simulink model "IFM_ModelComposer"  (R2024b)
settings: Solver=VariableStepAuto  StartTime=0.0  StopTime=2e-4  RelTol=1e-3
PreLoadFcn:
  | System
values from neighbouring files (symbols this model uses):
  Fs = 300e6    (= 300000000)    [IFM.m]    (also in System.m; SystemInput.m = p.Results.Fs)
  JustNoiseSamples = Fs*JustNoiseTime    (= 30000)    [IFM.m]    (also in System.m; SystemInput.m = Fs * 100e-6)
undefined symbols (not defined in the file or in its folder): IFM, Trial
libraries: hdlBasic x91, hdlDSPIP x2, vmcUtilities x1
settings Model: Creator=fsy  LastModifiedBy=fsy

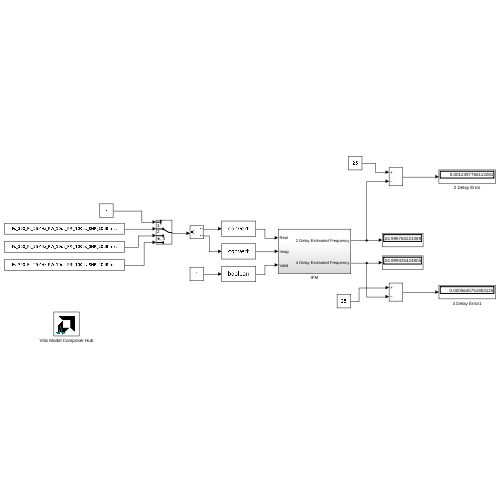
[thumbnail: Simulink's stored preview of the top-level diagram]
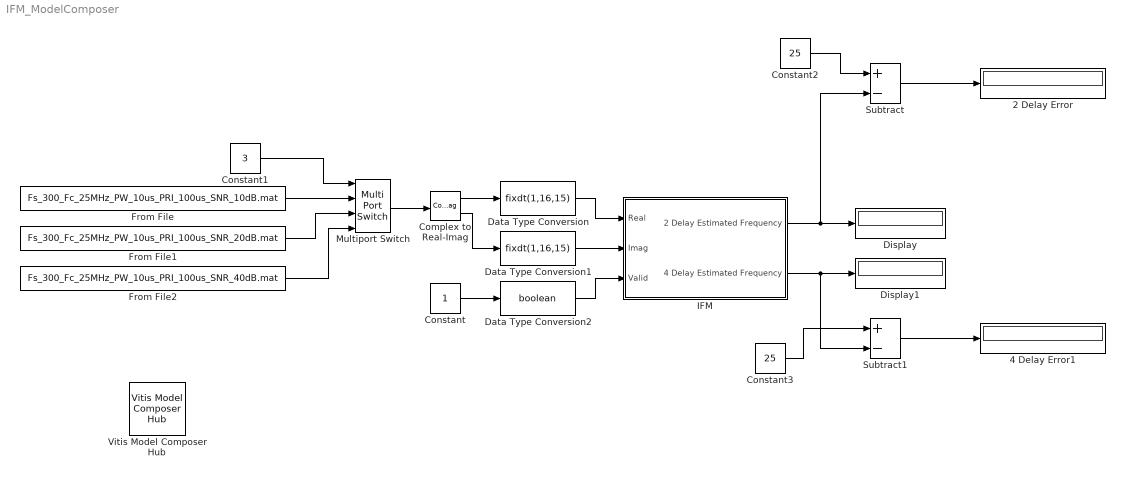
== system IFM_ModelComposer ==
  2 Delay Error : Display
  4 Delay Error1 : Display
  Complex to Real-Imag : ComplexToRealImag
  Constant : Constant  SampleTime=1/Fs
  Constant1 : Constant  Value=3  SampleTime=1/Fs
  Constant2 : Constant  Value=25  SampleTime=1/Fs
  Constant3 : Constant  Value=25  SampleTime=1/Fs
  Data Type Conversion : DataTypeConversion  OutDataTypeStr=fixdt(1,16,15)  RndMeth=Round
  Data Type Conversion1 : DataTypeConversion  OutDataTypeStr=fixdt(1,16,15)  RndMeth=Round
  Data Type Conversion2 : DataTypeConversion  OutDataTypeStr=boolean  RndMeth=Round
  Display : Display
  Display1 : Display
  From File : FromFile  FileName=Fs_300_Fc_25MHz_PW_10us_PRI_100us_SNR_10dB.mat  SampleTime=1/Fs
  From File1 : FromFile  FileName=Fs_300_Fc_25MHz_PW_10us_PRI_100us_SNR_20dB.mat  SampleTime=1/Fs
  From File2 : FromFile  FileName=Fs_300_Fc_25MHz_PW_10us_PRI_100us_SNR_40dB.mat  SampleTime=1/Fs
  IFM : Subsystem
  Multiport Switch : MultiPortSwitch  OutDataTypeStr=double  SaturateOnIntegerOverflow=off  InputSameDT=off
  Subtract : Sum  Inputs=+-
  Subtract1 : Sum  Inputs=+-
  Vitis Model Composer Hub : vmcUtilities/Vitis Model Composer Hub  Tag=genX  CodeGeneration=off  SubsystemName=IFM  BlockHierPath=Trial/IFM  CompilationType=HDLCompilation  SubsystemType=HDLNode  ExportTypeV2=IP Catalog  StartColumn=1  NumberOfColumns=1  TargetDirectory=./netlist\ip\IFM\src  exportDesign=off  analyzeDesign=on  validateDesignOnHw=off  ExportType=AI Engines  IpVendor=xilinx.com  IpLibrary=hls  IpVersion=1.0  IpHWLanguage=Verilog  AieCompilerOptions={}  AieSimulatorOptions={}  CreateTestbench=on  TestbenchStackSize=10  RunRtlSim=off  RunCSim=off  RunAieSim=off  AieSimTimeout=50000  RunAieSimProfiling=off  LaunchVitisAnalyzer=off  PlotOutput=off  RunX86Sim=off  X86SimTimeout=10  GenHwImage=off  GenLibadfXo=on  GenHwValidationCode=off  PlatformType=Not Specified  HwSystemType=Baremetal  HwValidationTarget=hw  ProjDevice=Zynq UltraScale+ ZCU102 Evaluation Board (xczu9eg-ffvb1156-2-e)  ProjDevicePart=xczu9eg-ffvb1156-2-e  AIEType=None  SamplePeriod=-1  ClockFrequency=200  DataPathParallelism=1  xilinxfamily=zynquplus  part=xczu9eg  speed=-2-e  package=ffvb1156  directory=./netlist\ip\IFM\src  testbench=off  incr_netlist=off  synthesis_tool=Vivado  clock_wrapper=Clock Enables  dbl_ovrd=According to Block Masks  dcm_input_clock_period=10  sysclk_period=1e9/Fs  simulink_period=1/Fs  eval_field=0  IPInfoJsonString="{\"DUTSubsystemName\":\"IFM\",\"HDLSubsystem\":{\"SubsystemName\":\"IFM\",\"IPName\":\"Subsystem\",\"IPLibrary\":\"VMC\",\"IPVendor\":\"User Company\",\"IPVersion\":\"1.0\",\"TargetDirectory\":\"./netlist\",\"SubsystemDir\":\"./netlist\\\\ip\\\\IFM\",\"FreqHz\":\"300000000\"},\"SubsystemTag\":\"HDLNode\"}"  LogFileName=C:\Users\fsydere\Workspace\IFM\Model Composer\netlist\model_composer.log  NThreads=4  IPConfigFile=C:\Users\fsydere\AppData\Local\Temp\vmctmp-13469454594715593076\Trial_ipconfig.json
  wires:
  Subtract/1 -> 2 Delay Error/1
  IFM/2(4 Delay Estimated Frequency) -> Subtract1/2, Display1/1
  IFM/1(2 Delay Estimated Frequency) -> Subtract/2, Display/1
  Data Type Conversion1/1 -> IFM/2(Imag)
  Data Type Conversion2/1 -> IFM/3(Valid)
  Data Type Conversion/1 -> IFM/1(Real)
  Complex to Real-Imag/2 -> Data Type Conversion1/1
  Constant/1 -> Data Type Conversion2/1
  Constant1/1 -> Multiport Switch/1
  Subtract1/1 -> 4 Delay Error1/1
  From File/1 -> Multiport Switch/2
  Multiport Switch/1 -> Complex to Real-Imag/1
  From File1/1 -> Multiport Switch/3
  Complex to Real-Imag/1 -> Data Type Conversion/1
  From File2/1 -> Multiport Switch/4
  Constant3/1 -> Subtract1/1
  Constant2/1 -> Subtract/1

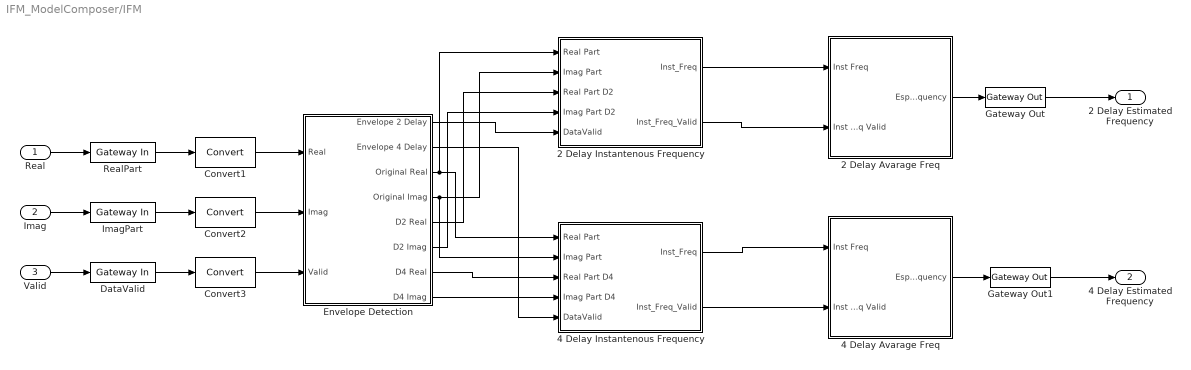
== system IFM_ModelComposer/IFM ==
  Real : Inport
  Imag : Inport  Port=2
  Valid : Inport  Port=3
  2 Delay Avarage Freq : Subsystem
  2 Delay Instantenous Frequency : Subsystem
  4 Delay Avarage Freq : Subsystem
  4 Delay Instantenous Frequency : Subsystem
  Convert1 : hdlBasic/Convert  gui_display_data_type=Fixed-point  arith_type="Signed  (2's comp)"  n_bits=16  bin_pt=15  float_type=Single  exp_bits=8  fraction_bits=24  quantization=Truncate  overflow=Wrap  en=off  latency=0  pipeline=off  XmcBlockStatus=1  maskContainerNames=group2  block_type=convert  block_config=sysgen:Convert_config  block_width=595  block_height=885
  Convert2 : hdlBasic/Convert  gui_display_data_type=Fixed-point  arith_type="Signed  (2's comp)"  n_bits=16  bin_pt=15  float_type=Single  exp_bits=8  fraction_bits=24  quantization=Truncate  overflow=Wrap  en=off  latency=0  pipeline=off  XmcBlockStatus=1  maskContainerNames=group2  block_type=convert  block_config=sysgen:Convert_config  block_width=595  block_height=885
  Convert3 : hdlBasic/Convert  gui_display_data_type=Boolean  arith_type=Boolean  n_bits=16  bin_pt=15  float_type=Single  exp_bits=8  fraction_bits=24  quantization=Truncate  overflow=Wrap  en=off  latency=0  pipeline=off  XmcBlockStatus=1  maskContainerNames=group2  block_type=convert  block_config=sysgen:Convert_config  block_width=595  block_height=885
  DataValid : hdlBasic/Gateway In  gui_display_data_type=Boolean  arith_type=Boolean  n_bits=16  bin_pt=15  preci_type=Single  exp_width=8  frac_width=24  rows=1  columns=1  quantization="Round  (unbiased: +/- Inf)"  overflow=Saturate  period=1/Fs  UseAsADC=off  ADCChannel='1'  interface=None  automatic_assignment=on  address_offset=hex2dec('00')  intf_name=''  intf_description=''  default_value=0  timing_constraint=None  locs_specified=off  LOCs={}  io_standard={}  inherit_from_input=off  hdl_port=on  XmcBlockStatus=1  maskContainerNames=group4  block_type=gatewayin  block_config=sysgen:gateway_in_config  block_width_w=590  block_height_w=620  block_width=640  block_height=850
  Envelope Detection : Subsystem
  Gateway Out : hdlBasic/Gateway Out  inherit_from_input=on  bool_to_boolean=off  hdl_port=off  rows=1  columns=1  UseAsDAC=off  DACChannel='1'  interface=None  automatic_assignment=on  address_offset=hex2dec('00')  intf_name=''  intf_description=''  timing_constraint=None  locs_specified=off  LOCs={}  io_standard={}  XmcBlockStatus=1  maskContainerNames=group4  block_type=gatewayout  block_config=sysgen:gateway_out_config  block_width_w=590  block_height_w=620  block_width=620  block_height=750
  Gateway Out1 : hdlBasic/Gateway Out  inherit_from_input=on  bool_to_boolean=off  hdl_port=off  rows=1  columns=1  UseAsDAC=off  DACChannel='1'  interface=None  automatic_assignment=on  address_offset=hex2dec('00')  intf_name=''  intf_description=''  timing_constraint=None  locs_specified=off  LOCs={}  io_standard={}  XmcBlockStatus=1  maskContainerNames=group4  block_type=gatewayout  block_config=sysgen:gateway_out_config  block_width_w=590  block_height_w=620  block_width=620  block_height=750
  ImagPart : hdlBasic/Gateway In  gui_display_data_type=Fixed-point  arith_type=Signed (2's comp)  n_bits=16  bin_pt=15  preci_type=Single  exp_width=8  frac_width=24  rows=1  columns=1  quantization=Truncate  overflow=Wrap  period=1/Fs  UseAsADC=off  ADCChannel='1'  interface=None  automatic_assignment=on  address_offset=hex2dec('00')  intf_name=''  intf_description=''  default_value=0  timing_constraint=None  locs_specified=off  LOCs={}  io_standard={}  inherit_from_input=off  hdl_port=on  XmcBlockStatus=1  maskContainerNames=group4  block_type=gatewayin  block_config=sysgen:gateway_in_config  block_width_w=590  block_height_w=620  block_width=640  block_height=850
  RealPart : hdlBasic/Gateway In  gui_display_data_type=Fixed-point  arith_type=Signed (2's comp)  n_bits=16  bin_pt=15  preci_type=Single  exp_width=8  frac_width=24  rows=1  columns=1  quantization=Truncate  overflow=Wrap  period=1/Fs  UseAsADC=off  ADCChannel='1'  interface=None  automatic_assignment=on  address_offset=hex2dec('00')  intf_name=''  intf_description=''  default_value=0  timing_constraint=None  locs_specified=off  LOCs={}  io_standard={}  inherit_from_input=off  hdl_port=on  XmcBlockStatus=1  maskContainerNames=group4  block_type=gatewayin  block_config=sysgen:gateway_in_config  block_width_w=590  block_height_w=620  block_width=640  block_height=850
  2 Delay Estimated Frequency : Outport
  4 Delay Estimated Frequency : Outport  Port=2
  wires:
  Real/1 -> RealPart/1
  Valid/1 -> DataValid/1
  Imag/1 -> ImagPart/1
  RealPart/1 -> Convert1/1
  ImagPart/1 -> Convert2/1
  Convert2/1 -> Envelope Detection/2(Imag)
  Convert1/1 -> Envelope Detection/1(Real)
  Envelope Detection/6(D2 Imag) -> 2 Delay Instantenous Frequency/4(Imag Part D2)
  DataValid/1 -> Convert3/1
  Convert3/1 -> Envelope Detection/3(Valid)
  Envelope Detection/1(Envelope 2 Delay) -> 2 Delay Instantenous Frequency/5(DataValid)
  Envelope Detection/5(D2 Real) -> 2 Delay Instantenous Frequency/3(Real Part D2)
  Envelope Detection/2(Envelope 4 Delay) -> 4 Delay Instantenous Frequency/5(DataValid)
  Envelope Detection/3(Original Real) -> 2 Delay Instantenous Frequency/1(Real Part), 4 Delay Instantenous Frequency/1(Real Part)
  Envelope Detection/4(Original Imag) -> 2 Delay Instantenous Frequency/2(Imag Part), 4 Delay Instantenous Frequency/2(Imag Part)
  Envelope Detection/7(D4 Real) -> 4 Delay Instantenous Frequency/3(Real Part D4)
  Envelope Detection/8(D4 Imag) -> 4 Delay Instantenous Frequency/4(Imag Part D4)
  2 Delay Instantenous Frequency/1(Inst_Freq) -> 2 Delay Avarage Freq/1(Inst Freq)
  2 Delay Instantenous Frequency/2(Inst_Freq_Valid) -> 2 Delay Avarage Freq/2(Inst Freq Valid)
  4 Delay Instantenous Frequency/1(Inst_Freq) -> 4 Delay Avarage Freq/1(Inst Freq)
  4 Delay Instantenous Frequency/2(Inst_Freq_Valid) -> 4 Delay Avarage Freq/2(Inst Freq Valid)
  4 Delay Avarage Freq/1(Espected Frequency) -> Gateway Out1/1
  2 Delay Avarage Freq/1(Espected Frequency) -> Gateway Out/1
  Gateway Out/1 -> 2 Delay Estimated Frequency/1
  Gateway Out1/1 -> 4 Delay Estimated Frequency/1

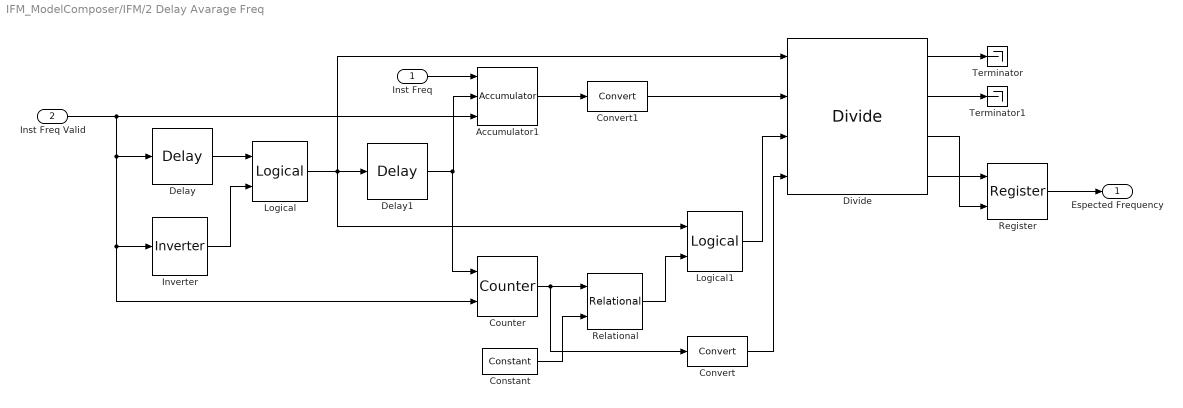
== system IFM_ModelComposer/IFM/2 Delay Avarage Freq ==
  Inst Freq : Inport
  Inst Freq Valid : Inport  Port=2
  Accumulator1 : hdlBasic/Accumulator  operation=Add  n_bits=64  overflow=Wrap  scale=1  rst=on  hasbypass=off  en=on  latency=1  msb_inp=100  msb=100  lsb=-100  use_behavioral_HDL=on  implementation=Fabric  XmcBlockStatus=1  maskContainerNames=group3  block_type=accum  block_config=sysgen:Accum_config  block_width=566  block_height=845
  Constant : hdlBasic/Constant  const=2  gui_display_data_type=Fixed-point  arith_type=Unsigned  n_bits=16  bin_pt=0  preci_type=Single  exp_width=8  frac_width=24  explicit_period=off  period=1  XmcBlockStatus=1  maskContainerNames=tabcontainer1  block_type=constant  block_config=sysgen:Constant_config
  Convert : hdlBasic/Convert  gui_display_data_type=Fixed-point  arith_type="Signed  (2's comp)"  n_bits=64  bin_pt=26  float_type=Single  exp_bits=8  fraction_bits=24  quantization=Truncate  overflow=Wrap  en=off  latency=0  pipeline=off  XmcBlockStatus=1  maskContainerNames=group2  block_type=convert  block_config=sysgen:Convert_config  block_width=595  block_height=885
  Convert1 : hdlBasic/Convert  gui_display_data_type=Fixed-point  arith_type="Signed  (2's comp)"  n_bits=64  bin_pt=26  float_type=Single  exp_bits=8  fraction_bits=24  quantization=Truncate  overflow=Wrap  en=off  latency=0  pipeline=off  XmcBlockStatus=1  maskContainerNames=group2  block_type=convert  block_config=sysgen:Convert_config  block_width=595  block_height=885
  Counter : hdlBasic/Counter  cnt_type=Free running  cnt_to=Inf  operation=Up  start_count=0  cnt_by_val=1  arith_type=Unsigned  n_bits=16  bin_pt=0  load_pin=off  rst=on  en=on  explicit_period=Explicit  period=1/Fs  use_behavioral_HDL=off  implementation=Fabric  XmcBlockStatus=1  maskContainerNames=group1  block_type=counter  block_config=sysgen:Counter_config  block_width=531  block_height=1023
  Delay : hdlBasic/Delay  rst=off  en=off  latency=1  reg_retiming=off  XmcBlockStatus=1  maskContainerNames=group1  block_type=delay  block_config=sysgen:Delay_config
  Delay1 : hdlBasic/Delay  rst=off  en=off  latency=1  reg_retiming=off  XmcBlockStatus=1  maskContainerNames=group1  block_type=delay  block_config=sysgen:Delay_config
  Divide : hdlBasic/Divide  flow_control=Blocking  axi_optimize_goal=Resources  algorithm_type=High_Radix  fractional_width=26  latency=1  rate=1  has_a_tlast=off  has_a_tuser=off  has_b_tlast=off  has_b_tuser=off  en=off  has_result_tready=off  result_tlast_behv=Pass_A_TLAST  has_underflow=off  has_overflow=off  has_invalid_op=off  has_divide_by_zero=off  fpo_op_type=mergeddivide  XmcBlockStatus=1  maskContainerNames=tabcontainer1  block_type=divide  block_config=sysgen:FPOBlockDescriptor_config
  Inverter : hdlBasic/Inverter  en=off  latency=0  XmcBlockStatus=1  maskContainerNames=group2  block_type=inv  block_config=sysgen:Inverter_config
  Logical : hdlBasic/Logical  logical_function=AND  inputs=2  en=off  latency=0  precision=Full  arith_type=Unsigned  n_bits=16  bin_pt=0  align_bp=on  overflow=[]  quantization=[]  XmcBlockStatus=1  maskContainerNames=tabcontainer1  block_type=logical  block_config=sysgen:Logical_config
  Logical1 : hdlBasic/Logical  logical_function=AND  inputs=2  en=off  latency=0  precision=Full  arith_type=Unsigned  n_bits=16  bin_pt=0  align_bp=on  overflow=[]  quantization=[]  XmcBlockStatus=1  maskContainerNames=tabcontainer1  block_type=logical  block_config=sysgen:Logical_config
  Register : hdlBasic/Register  init=0  rst=off  en=on  XmcBlockStatus=1  maskContainerNames=tabcontainer1  block_type=register  block_config=sysgen:Register_config
  Relational : hdlBasic/Relational  mode=a>b  op_type=Bool  en=off  latency=0  XmcBlockStatus=1  maskContainerNames=tabcontainer1  block_type=relational  block_config=sysgen:Relational_config
  Terminator : Terminator
  Terminator1 : Terminator
  Espected Frequency : Outport
  wires:
  Register/1 -> Espected Frequency/1
  Divide/4 -> Register/1
  Divide/2 -> Terminator1/1
  Inst Freq Valid/1 -> Inverter/1, Counter/2, Delay/1, Accumulator1/3
  Inverter/1 -> Logical/2
  Logical/1 -> Delay1/1, Logical1/1, Divide/1
  Divide/1 -> Terminator/1
  Accumulator1/1 -> Convert1/1
  Delay1/1 -> Counter/1, Accumulator1/2
  Counter/1 -> Relational/1, Convert/1
  Delay/1 -> Logical/1
  Constant/1 -> Relational/2
  Inst Freq/1 -> Accumulator1/1
  Convert1/1 -> Divide/2
  Convert/1 -> Divide/4
  Divide/3 -> Register/2
  Relational/1 -> Logical1/2
  Logical1/1 -> Divide/3

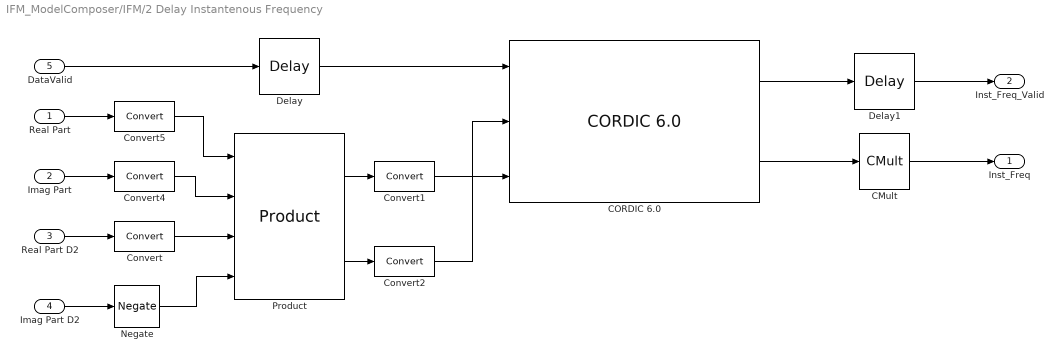
== system IFM_ModelComposer/IFM/2 Delay Instantenous Frequency ==
  Real Part : Inport
  Imag Part : Inport  Port=2
  Real Part D2 : Inport  Port=3
  Imag Part D2 : Inport  Port=4
  DataValid : Inport  Port=5
  CMult : hdlBasic/CMult  const=Fs/(2*pi*2*1e6)  gui_display_data_type=Fixed-point  const_n_bits=20  const_bin_pt=13  float_type=Single  exp_bits=8  fraction_bits=24  en=off  latency=1  precision=Full  arith_type="Signed  (2's comp)"  n_bits=16  bin_pt=14  quantization=Truncate  overflow=Wrap  use_behavioral_HDL=off  mem_type=Distributed RAM  pipeline=off  XmcBlockStatus=1  maskContainerNames=tabcontainer1  block_type=cmult  block_config=sysgen:CMult_config
      settings: infoedit=[]
  CORDIC 6.0 : hdlDSPIP/CORDIC 6.0   functional_selection=Arc_Tan  architectural_configuration=Parallel  pipelining_mode=Maximum  data_format=SignedFraction  phase_format=Radians  input_width=33  output_width=16  round_mode=Truncate  iterations=0  precision=0  compensation_scaling=No_Scale_Compensation  coarse_rotation=on  aclken=off  aresetn=off  out_tready=off  cartesian_has_tuser=off  cartesian_has_tlast=off  cartesian_tuser_width=1  phase_has_tuser=off  phase_has_tlast=off  phase_tuser_width=1  out_tlast_behv=Null  flow_control=NonBlocking  optimize_goal=Resources  trim_axipin_name=on  simulation_type=hybrid_sim  simulation_model=sysgen:cordic_v6_0  data_path_portlist={'s_axis_cartesian_tdata_imag', 's_axis_cartesian_tdata_real', 's_axis_phase_tdata_phase', 'm_axis_dout_tdata_imag', 'm_axis_dout_tdata_real', 'm_axis_dout_tdata_phase','m_axis_dout_tdata'}  ip_name=CORDIC  ip_version=6.0  dsptool_ready=true  ipcore_usecache=true  ipcore_useipmodelcache=true  wrapper_available=true  port_translation_map={ 'aclken' => 'en', 'aresetn' => 'rst' }  XmcBlockStatus=1  maskContainerNames=group15  block_type=cordic_v6_0  block_config=sysgen:rodinimport_config  block_width=800
  Convert : hdlBasic/Convert  gui_display_data_type=Fixed-point  arith_type="Signed  (2's comp)"  n_bits=17  bin_pt=15  float_type=Single  exp_bits=8  fraction_bits=24  quantization=Truncate  overflow=Wrap  en=off  latency=1  pipeline=off  XmcBlockStatus=1  maskContainerNames=group2  block_type=convert  block_config=sysgen:Convert_config  block_width=595  block_height=885
  Convert1 : hdlBasic/Convert  gui_display_data_type=Fixed-point  arith_type="Signed  (2's comp)"  n_bits=35  bin_pt=33  float_type=Single  exp_bits=8  fraction_bits=24  quantization=Truncate  overflow=Wrap  en=off  latency=0  pipeline=off  XmcBlockStatus=1  maskContainerNames=group2  block_type=convert  block_config=sysgen:Convert_config  block_width=595  block_height=885
  Convert2 : hdlBasic/Convert  gui_display_data_type=Fixed-point  arith_type="Signed  (2's comp)"  n_bits=35  bin_pt=33  float_type=Single  exp_bits=8  fraction_bits=24  quantization=Truncate  overflow=Wrap  en=off  latency=0  pipeline=off  XmcBlockStatus=1  maskContainerNames=group2  block_type=convert  block_config=sysgen:Convert_config  block_width=595  block_height=885
  Convert4 : hdlBasic/Convert  gui_display_data_type=Fixed-point  arith_type="Signed  (2's comp)"  n_bits=17  bin_pt=15  float_type=Single  exp_bits=8  fraction_bits=24  quantization=Truncate  overflow=Wrap  en=off  latency=1  pipeline=off  XmcBlockStatus=1  maskContainerNames=group2  block_type=convert  block_config=sysgen:Convert_config  block_width=595  block_height=885
  Convert5 : hdlBasic/Convert  gui_display_data_type=Fixed-point  arith_type="Signed  (2's comp)"  n_bits=17  bin_pt=15  float_type=Single  exp_bits=8  fraction_bits=24  quantization=Truncate  overflow=Wrap  en=off  latency=1  pipeline=off  XmcBlockStatus=1  maskContainerNames=group2  block_type=convert  block_config=sysgen:Convert_config  block_width=595  block_height=885
  Delay : hdlBasic/Delay  rst=off  en=off  latency=5  reg_retiming=off  XmcBlockStatus=1  maskContainerNames=group1  block_type=delay  block_config=sysgen:Delay_config
  Delay1 : hdlBasic/Delay  rst=off  en=off  latency=1  reg_retiming=off  XmcBlockStatus=1  maskContainerNames=group1  block_type=delay  block_config=sysgen:Delay_config
  Negate : hdlBasic/Negate  precision=User Defined  arith_type="Signed  (2's comp)"  n_bits=17  bin_pt=15  quantization=Truncate  overflow=Wrap  en=off  latency=1  XmcBlockStatus=1  maskContainerNames=tabcontainer1  block_type=negate  block_config=sysgen:Negate_config
  Product : hdlBasic/Product  complex_multiplier=on  optimizegoal=Performance  simulation_type=fast_sim  simulation_model=sysgen:product_macro  XmcBlockStatus=1  maskContainerNames=<empty>  block_type=product_macro  block_config=sysgen:ProductMacro_config
  Inst_Freq : Outport
  Inst_Freq_Valid : Outport  Port=2
  wires:
  Real Part/1 -> Convert5/1
  Imag Part/1 -> Convert4/1
  Real Part D2/1 -> Convert/1
  Imag Part D2/1 -> Negate/1
  DataValid/1 -> Delay/1
  Convert/1 -> Product/3
  Convert4/1 -> Product/2
  Convert5/1 -> Product/1
  Negate/1 -> Product/4
  Delay/1 -> CORDIC 6.0/1
  CORDIC 6.0/2 -> CMult/1
  CORDIC 6.0/1 -> Delay1/1
  Product/1 -> Convert1/1
  Product/2 -> Convert2/1
  Convert1/1 -> CORDIC 6.0/3
  Convert2/1 -> CORDIC 6.0/2
  CMult/1 -> Inst_Freq/1
  Delay1/1 -> Inst_Freq_Valid/1

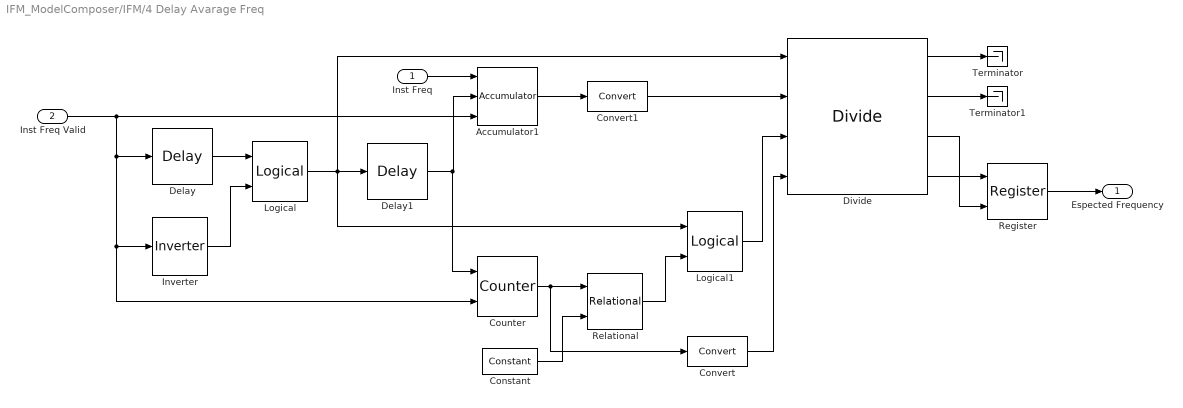
== system IFM_ModelComposer/IFM/4 Delay Avarage Freq ==
  Inst Freq : Inport
  Inst Freq Valid : Inport  Port=2
  Accumulator1 : hdlBasic/Accumulator  operation=Add  n_bits=64  overflow=Wrap  scale=1  rst=on  hasbypass=off  en=on  latency=1  msb_inp=100  msb=100  lsb=-100  use_behavioral_HDL=on  implementation=Fabric  XmcBlockStatus=1  maskContainerNames=group3  block_type=accum  block_config=sysgen:Accum_config  block_width=566  block_height=845
  Constant : hdlBasic/Constant  const=4  gui_display_data_type=Fixed-point  arith_type=Unsigned  n_bits=16  bin_pt=0  preci_type=Single  exp_width=8  frac_width=24  explicit_period=off  period=1  XmcBlockStatus=1  maskContainerNames=tabcontainer1  block_type=constant  block_config=sysgen:Constant_config
  Convert : hdlBasic/Convert  gui_display_data_type=Fixed-point  arith_type="Signed  (2's comp)"  n_bits=64  bin_pt=26  float_type=Single  exp_bits=8  fraction_bits=24  quantization=Truncate  overflow=Wrap  en=off  latency=0  pipeline=off  XmcBlockStatus=1  maskContainerNames=group2  block_type=convert  block_config=sysgen:Convert_config  block_width=595  block_height=885
  Convert1 : hdlBasic/Convert  gui_display_data_type=Fixed-point  arith_type="Signed  (2's comp)"  n_bits=64  bin_pt=26  float_type=Single  exp_bits=8  fraction_bits=24  quantization=Truncate  overflow=Wrap  en=off  latency=0  pipeline=off  XmcBlockStatus=1  maskContainerNames=group2  block_type=convert  block_config=sysgen:Convert_config  block_width=595  block_height=885
  Counter : hdlBasic/Counter  cnt_type=Free running  cnt_to=Inf  operation=Up  start_count=0  cnt_by_val=1  arith_type=Unsigned  n_bits=16  bin_pt=0  load_pin=off  rst=on  en=on  explicit_period=Explicit  period=1/Fs  use_behavioral_HDL=off  implementation=Fabric  XmcBlockStatus=1  maskContainerNames=group1  block_type=counter  block_config=sysgen:Counter_config  block_width=531  block_height=1023
  Delay : hdlBasic/Delay  rst=off  en=off  latency=1  reg_retiming=off  XmcBlockStatus=1  maskContainerNames=group1  block_type=delay  block_config=sysgen:Delay_config
  Delay1 : hdlBasic/Delay  rst=off  en=off  latency=1  reg_retiming=off  XmcBlockStatus=1  maskContainerNames=group1  block_type=delay  block_config=sysgen:Delay_config
  Divide : hdlBasic/Divide  flow_control=Blocking  axi_optimize_goal=Resources  algorithm_type=High_Radix  fractional_width=26  latency=1  rate=1  has_a_tlast=off  has_a_tuser=off  has_b_tlast=off  has_b_tuser=off  en=off  has_result_tready=off  result_tlast_behv=Pass_A_TLAST  has_underflow=off  has_overflow=off  has_invalid_op=off  has_divide_by_zero=off  fpo_op_type=mergeddivide  XmcBlockStatus=1  maskContainerNames=tabcontainer1  block_type=divide  block_config=sysgen:FPOBlockDescriptor_config
  Inverter : hdlBasic/Inverter  en=off  latency=0  XmcBlockStatus=1  maskContainerNames=group2  block_type=inv  block_config=sysgen:Inverter_config
  Logical : hdlBasic/Logical  logical_function=AND  inputs=2  en=off  latency=0  precision=Full  arith_type=Unsigned  n_bits=16  bin_pt=0  align_bp=on  overflow=[]  quantization=[]  XmcBlockStatus=1  maskContainerNames=tabcontainer1  block_type=logical  block_config=sysgen:Logical_config
  Logical1 : hdlBasic/Logical  logical_function=AND  inputs=2  en=off  latency=0  precision=Full  arith_type=Unsigned  n_bits=16  bin_pt=0  align_bp=on  overflow=[]  quantization=[]  XmcBlockStatus=1  maskContainerNames=tabcontainer1  block_type=logical  block_config=sysgen:Logical_config
  Register : hdlBasic/Register  init=0  rst=off  en=on  XmcBlockStatus=1  maskContainerNames=tabcontainer1  block_type=register  block_config=sysgen:Register_config
  Relational : hdlBasic/Relational  mode=a>b  op_type=Bool  en=off  latency=0  XmcBlockStatus=1  maskContainerNames=tabcontainer1  block_type=relational  block_config=sysgen:Relational_config
  Terminator : Terminator
  Terminator1 : Terminator
  Espected Frequency : Outport
  wires:
  Register/1 -> Espected Frequency/1
  Divide/4 -> Register/1
  Divide/2 -> Terminator1/1
  Inst Freq Valid/1 -> Inverter/1, Counter/2, Delay/1, Accumulator1/3
  Inverter/1 -> Logical/2
  Logical/1 -> Delay1/1, Logical1/1, Divide/1
  Divide/1 -> Terminator/1
  Accumulator1/1 -> Convert1/1
  Delay1/1 -> Counter/1, Accumulator1/2
  Counter/1 -> Relational/1, Convert/1
  Delay/1 -> Logical/1
  Constant/1 -> Relational/2
  Inst Freq/1 -> Accumulator1/1
  Convert1/1 -> Divide/2
  Convert/1 -> Divide/4
  Divide/3 -> Register/2
  Relational/1 -> Logical1/2
  Logical1/1 -> Divide/3

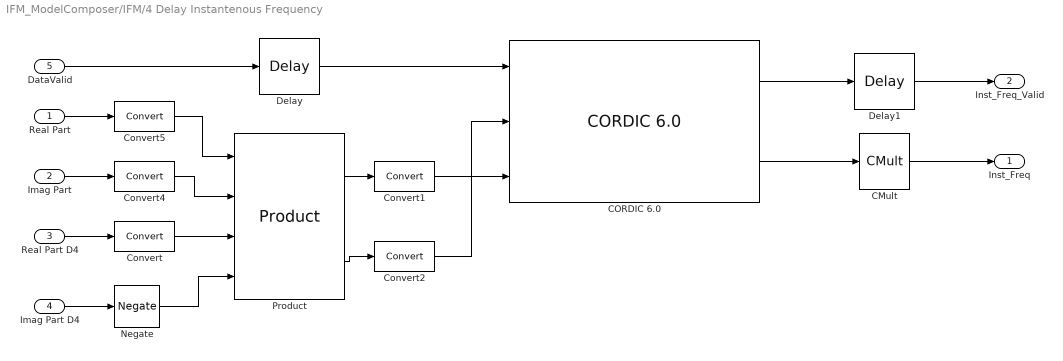
== system IFM_ModelComposer/IFM/4 Delay Instantenous Frequency ==
  Real Part : Inport
  Imag Part : Inport  Port=2
  Real Part D4 : Inport  Port=3
  Imag Part D4 : Inport  Port=4
  DataValid : Inport  Port=5
  CMult : hdlBasic/CMult  const=Fs/(2*pi*4*1e6)  gui_display_data_type=Fixed-point  const_n_bits=20  const_bin_pt=13  float_type=Single  exp_bits=8  fraction_bits=24  en=off  latency=1  precision=Full  arith_type="Signed  (2's comp)"  n_bits=16  bin_pt=14  quantization=Truncate  overflow=Wrap  use_behavioral_HDL=off  mem_type=Distributed RAM  pipeline=off  XmcBlockStatus=1  maskContainerNames=tabcontainer1  block_type=cmult  block_config=sysgen:CMult_config
      settings: infoedit=[]
  CORDIC 6.0 : hdlDSPIP/CORDIC 6.0   functional_selection=Arc_Tan  architectural_configuration=Parallel  pipelining_mode=Maximum  data_format=SignedFraction  phase_format=Radians  input_width=33  output_width=16  round_mode=Truncate  iterations=0  precision=0  compensation_scaling=No_Scale_Compensation  coarse_rotation=on  aclken=off  aresetn=off  out_tready=off  cartesian_has_tuser=off  cartesian_has_tlast=off  cartesian_tuser_width=1  phase_has_tuser=off  phase_has_tlast=off  phase_tuser_width=1  out_tlast_behv=Null  flow_control=NonBlocking  optimize_goal=Resources  trim_axipin_name=on  simulation_type=hybrid_sim  simulation_model=sysgen:cordic_v6_0  data_path_portlist={'s_axis_cartesian_tdata_imag', 's_axis_cartesian_tdata_real', 's_axis_phase_tdata_phase', 'm_axis_dout_tdata_imag', 'm_axis_dout_tdata_real', 'm_axis_dout_tdata_phase','m_axis_dout_tdata'}  ip_name=CORDIC  ip_version=6.0  dsptool_ready=true  ipcore_usecache=true  ipcore_useipmodelcache=true  wrapper_available=true  port_translation_map={ 'aclken' => 'en', 'aresetn' => 'rst' }  XmcBlockStatus=1  maskContainerNames=group15  block_type=cordic_v6_0  block_config=sysgen:rodinimport_config  block_width=800
  Convert : hdlBasic/Convert  gui_display_data_type=Fixed-point  arith_type="Signed  (2's comp)"  n_bits=17  bin_pt=15  float_type=Single  exp_bits=8  fraction_bits=24  quantization=Truncate  overflow=Wrap  en=off  latency=1  pipeline=off  XmcBlockStatus=1  maskContainerNames=group2  block_type=convert  block_config=sysgen:Convert_config  block_width=595  block_height=885
  Convert1 : hdlBasic/Convert  gui_display_data_type=Fixed-point  arith_type="Signed  (2's comp)"  n_bits=35  bin_pt=33  float_type=Single  exp_bits=8  fraction_bits=24  quantization=Truncate  overflow=Wrap  en=off  latency=0  pipeline=off  XmcBlockStatus=1  maskContainerNames=group2  block_type=convert  block_config=sysgen:Convert_config  block_width=595  block_height=885
  Convert2 : hdlBasic/Convert  gui_display_data_type=Fixed-point  arith_type="Signed  (2's comp)"  n_bits=35  bin_pt=33  float_type=Single  exp_bits=8  fraction_bits=24  quantization=Truncate  overflow=Wrap  en=off  latency=0  pipeline=off  XmcBlockStatus=1  maskContainerNames=group2  block_type=convert  block_config=sysgen:Convert_config  block_width=595  block_height=885
  Convert4 : hdlBasic/Convert  gui_display_data_type=Fixed-point  arith_type="Signed  (2's comp)"  n_bits=17  bin_pt=15  float_type=Single  exp_bits=8  fraction_bits=24  quantization=Truncate  overflow=Wrap  en=off  latency=1  pipeline=off  XmcBlockStatus=1  maskContainerNames=group2  block_type=convert  block_config=sysgen:Convert_config  block_width=595  block_height=885
  Convert5 : hdlBasic/Convert  gui_display_data_type=Fixed-point  arith_type="Signed  (2's comp)"  n_bits=17  bin_pt=15  float_type=Single  exp_bits=8  fraction_bits=24  quantization=Truncate  overflow=Wrap  en=off  latency=1  pipeline=off  XmcBlockStatus=1  maskContainerNames=group2  block_type=convert  block_config=sysgen:Convert_config  block_width=595  block_height=885
  Delay : hdlBasic/Delay  rst=off  en=off  latency=5  reg_retiming=off  XmcBlockStatus=1  maskContainerNames=group1  block_type=delay  block_config=sysgen:Delay_config
  Delay1 : hdlBasic/Delay  rst=off  en=off  latency=1  reg_retiming=off  XmcBlockStatus=1  maskContainerNames=group1  block_type=delay  block_config=sysgen:Delay_config
  Negate : hdlBasic/Negate  precision=User Defined  arith_type="Signed  (2's comp)"  n_bits=17  bin_pt=15  quantization=Truncate  overflow=Wrap  en=off  latency=1  XmcBlockStatus=1  maskContainerNames=tabcontainer1  block_type=negate  block_config=sysgen:Negate_config
  Product : hdlBasic/Product  complex_multiplier=on  optimizegoal=Performance  simulation_type=fast_sim  simulation_model=sysgen:product_macro  XmcBlockStatus=1  maskContainerNames=<empty>  block_type=product_macro  block_config=sysgen:ProductMacro_config
  Inst_Freq : Outport
  Inst_Freq_Valid : Outport  Port=2
  wires:
  Real Part/1 -> Convert5/1
  Imag Part/1 -> Convert4/1
  Real Part D4/1 -> Convert/1
  Imag Part D4/1 -> Negate/1
  DataValid/1 -> Delay/1
  Convert/1 -> Product/3
  Convert4/1 -> Product/2
  Convert5/1 -> Product/1
  Negate/1 -> Product/4
  Delay/1 -> CORDIC 6.0/1
  CORDIC 6.0/2 -> CMult/1
  CORDIC 6.0/1 -> Delay1/1
  Product/1 -> Convert1/1
  Product/2 -> Convert2/1
  Convert1/1 -> CORDIC 6.0/3
  Convert2/1 -> CORDIC 6.0/2
  CMult/1 -> Inst_Freq/1
  Delay1/1 -> Inst_Freq_Valid/1

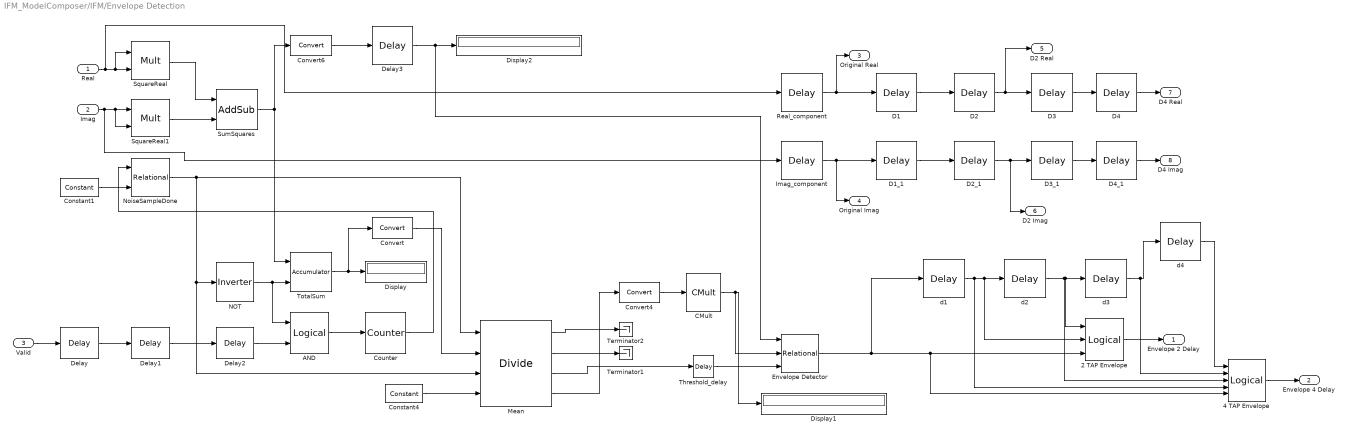
== system IFM_ModelComposer/IFM/Envelope Detection ==
  Real : Inport
  Imag : Inport  Port=2
  Valid : Inport  Port=3
  2 TAP Envelope : hdlBasic/Logical  logical_function=AND  inputs=3  en=off  latency=0  precision=Full  arith_type=Unsigned  n_bits=16  bin_pt=0  align_bp=on  overflow=[]  quantization=[]  XmcBlockStatus=1  maskContainerNames=tabcontainer1  block_type=logical  block_config=sysgen:Logical_config
  4 TAP Envelope : hdlBasic/Logical  logical_function=AND  inputs=5  en=off  latency=0  precision=Full  arith_type=Unsigned  n_bits=16  bin_pt=0  align_bp=on  overflow=[]  quantization=[]  XmcBlockStatus=1  maskContainerNames=tabcontainer1  block_type=logical  block_config=sysgen:Logical_config
  AND : hdlBasic/Logical  logical_function=AND  inputs=2  en=off  latency=0  precision=Full  arith_type=Unsigned  n_bits=16  bin_pt=0  align_bp=on  overflow=[]  quantization=[]  XmcBlockStatus=1  maskContainerNames=tabcontainer1  block_type=logical  block_config=sysgen:Logical_config
  CMult : hdlBasic/CMult  const=4  gui_display_data_type=Fixed-point  const_n_bits=48  const_bin_pt=30  float_type=Single  exp_bits=8  fraction_bits=24  en=off  latency=1  precision=Full  arith_type="Signed  (2's comp)"  n_bits=16  bin_pt=14  quantization=Truncate  overflow=Wrap  use_behavioral_HDL=off  mem_type=Distributed RAM  pipeline=off  XmcBlockStatus=1  maskContainerNames=tabcontainer1  block_type=cmult  block_config=sysgen:CMult_config
      settings: infoedit=[]
  Constant1 : hdlBasic/Constant  const=JustNoiseSamples-1  gui_display_data_type=Fixed-point  arith_type=Unsigned  n_bits=15  bin_pt=0  preci_type=Single  exp_width=8  frac_width=24  explicit_period=off  period=1  XmcBlockStatus=1  maskContainerNames=tabcontainer1  block_type=constant  block_config=sysgen:Constant_config
  Constant4 : hdlBasic/Constant  const=JustNoiseSamples/2  gui_display_data_type=Fixed-point  arith_type=Signed (2's comp)  n_bits=49  bin_pt=30  preci_type=Single  exp_width=8  frac_width=24  explicit_period=off  period=1  XmcBlockStatus=1  maskContainerNames=tabcontainer1  block_type=constant  block_config=sysgen:Constant_config
  Convert : hdlBasic/Convert  gui_display_data_type=Fixed-point  arith_type="Signed  (2's comp)"  n_bits=48  bin_pt=30  float_type=Single  exp_bits=8  fraction_bits=24  quantization="Round  (unbiased: +/- Inf)"  overflow=Saturate  en=off  latency=0  pipeline=off  XmcBlockStatus=1  maskContainerNames=group2  block_type=convert  block_config=sysgen:Convert_config  block_width=595  block_height=885
  Convert4 : hdlBasic/Convert  gui_display_data_type=Fixed-point  arith_type="Signed  (2's comp)"  n_bits=48  bin_pt=30  float_type=Single  exp_bits=8  fraction_bits=24  quantization="Round  (unbiased: +/- Inf)"  overflow=Saturate  en=off  latency=0  pipeline=off  XmcBlockStatus=1  maskContainerNames=group2  block_type=convert  block_config=sysgen:Convert_config  block_width=595  block_height=885
  Convert6 : hdlBasic/Convert  gui_display_data_type=Fixed-point  arith_type="Signed  (2's comp)"  n_bits=48  bin_pt=30  float_type=Single  exp_bits=8  fraction_bits=24  quantization="Round  (unbiased: +/- Inf)"  overflow=Saturate  en=off  latency=0  pipeline=off  XmcBlockStatus=1  maskContainerNames=group2  block_type=convert  block_config=sysgen:Convert_config  block_width=595  block_height=885
  Counter : hdlBasic/Counter  cnt_type=Count limited  cnt_to=JustNoiseSamples-1  operation=Up  start_count=0  cnt_by_val=1  arith_type=Unsigned  n_bits=15  bin_pt=0  load_pin=off  rst=off  en=on  explicit_period=Explicit  period=1/Fs  use_behavioral_HDL=off  implementation=Fabric  XmcBlockStatus=1  maskContainerNames=group1  block_type=counter  block_config=sysgen:Counter_config  block_width=531  block_height=1023
  D{1..4} (4 alike) : hdlBasic/Delay  rst=off  en=off  latency=1  reg_retiming=off  XmcBlockStatus=1  maskContainerNames=group1  block_type=delay  block_config=sysgen:Delay_config
  D1_1 : hdlBasic/Delay  rst=off  en=off  latency=1  reg_retiming=off  XmcBlockStatus=1  maskContainerNames=group1  block_type=delay  block_config=sysgen:Delay_config
  D2_1 : hdlBasic/Delay  rst=off  en=off  latency=1  reg_retiming=off  XmcBlockStatus=1  maskContainerNames=group1  block_type=delay  block_config=sysgen:Delay_config
  D3_1 : hdlBasic/Delay  rst=off  en=off  latency=1  reg_retiming=off  XmcBlockStatus=1  maskContainerNames=group1  block_type=delay  block_config=sysgen:Delay_config
  D4_1 : hdlBasic/Delay  rst=off  en=off  latency=1  reg_retiming=off  XmcBlockStatus=1  maskContainerNames=group1  block_type=delay  block_config=sysgen:Delay_config
  Delay : hdlBasic/Delay  rst=off  en=off  latency=3  reg_retiming=on  XmcBlockStatus=1  maskContainerNames=group1  block_type=delay  block_config=sysgen:Delay_config
  Delay1 : hdlBasic/Delay  rst=off  en=off  latency=1  reg_retiming=on  XmcBlockStatus=1  maskContainerNames=group1  block_type=delay  block_config=sysgen:Delay_config
  Delay2 : hdlBasic/Delay  rst=off  en=off  latency=1  reg_retiming=on  XmcBlockStatus=1  maskContainerNames=group1  block_type=delay  block_config=sysgen:Delay_config
  Delay3 : hdlBasic/Delay  rst=off  en=off  latency=3  reg_retiming=off  XmcBlockStatus=1  maskContainerNames=group1  block_type=delay  block_config=sysgen:Delay_config
  Display : Display
  Display1 : Display
  Display2 : Display
  Envelope Detector : hdlBasic/Relational  mode=a>=b  op_type=Bool  en=on  latency=1  XmcBlockStatus=1  maskContainerNames=tabcontainer1  block_type=relational  block_config=sysgen:Relational_config
  Imag_component : hdlBasic/Delay  rst=off  en=off  latency=8  reg_retiming=off  XmcBlockStatus=1  maskContainerNames=group1  block_type=delay  block_config=sysgen:Delay_config
  Mean : hdlBasic/Divide  flow_control=Blocking  axi_optimize_goal=Resources  algorithm_type=Radix2  fractional_width=30  latency=1  rate=1  has_a_tlast=off  has_a_tuser=off  has_b_tlast=off  has_b_tuser=off  en=off  has_result_tready=off  result_tlast_behv=Pass_A_TLAST  has_underflow=off  has_overflow=off  has_invalid_op=off  has_divide_by_zero=off  fpo_op_type=mergeddivide  XmcBlockStatus=1  maskContainerNames=tabcontainer1  block_type=divide  block_config=sysgen:FPOBlockDescriptor_config
  NOT : hdlBasic/Inverter  en=off  latency=0  XmcBlockStatus=1  maskContainerNames=group2  block_type=inv  block_config=sysgen:Inverter_config
  NoiseSampleDone : hdlBasic/Relational  mode=a=b  op_type=Bool  en=off  latency=0  XmcBlockStatus=1  maskContainerNames=tabcontainer1  block_type=relational  block_config=sysgen:Relational_config
  Real_component : hdlBasic/Delay  rst=off  en=off  latency=8  reg_retiming=off  XmcBlockStatus=1  maskContainerNames=group1  block_type=delay  block_config=sysgen:Delay_config
  SquareReal : hdlBasic/Mult  precision=User Defined  arith_type="Signed  (2's comp)"  n_bits=32  bin_pt=30  quantization="Round  (unbiased: +/- Inf)"  overflow=Saturate  en=off  latency=3  opt_float=off  fp_mult_usage=No Usage  use_behavioral_HDL=on  opt=Speed  use_embedded=on  optimum_pipeline=off  pipeline=on  use_rpm=on  placement_style=Triangular  XmcBlockStatus=1  maskContainerNames=group1  block_type=mult  block_config=sysgen:Mult_config  block_width=598  block_height=876
  SquareReal1 : hdlBasic/Mult  precision=User Defined  arith_type="Signed  (2's comp)"  n_bits=32  bin_pt=30  quantization="Round  (unbiased: +/- Inf)"  overflow=Saturate  en=off  latency=3  opt_float=off  fp_mult_usage=No Usage  use_behavioral_HDL=on  opt=Speed  use_embedded=on  optimum_pipeline=off  pipeline=on  use_rpm=on  placement_style=Triangular  XmcBlockStatus=1  maskContainerNames=group1  block_type=mult  block_config=sysgen:Mult_config  block_width=598  block_height=876
  SumSquares : hdlBasic/AddSub  mode=Addition  use_carryin=off  use_carryout=off  en=off  latency=1  precision=User Defined  arith_type=Unsigned  n_bits=32  bin_pt=30  quantization=Truncate  overflow=Wrap  use_behavioral_HDL=on  hw_selection=Fabric  pipelined=off  XmcBlockStatus=1  maskContainerNames=tabcontainer1  block_type=addsub  block_config=sysgen:Addsub_config
  Terminator1 : Terminator
  Terminator2 : Terminator
  Threshold_delay : hdlBasic/Delay  rst=off  en=off  latency=1  reg_retiming=off  XmcBlockStatus=1  maskContainerNames=group1  block_type=delay  block_config=sysgen:Delay_config
  TotalSum : hdlBasic/Accumulator  operation=Add  n_bits=48  overflow=Wrap  scale=1  rst=off  hasbypass=off  en=on  latency=1  msb_inp=32  msb=48  lsb=-30  use_behavioral_HDL=on  implementation=Fabric  XmcBlockStatus=1  maskContainerNames=group3  block_type=accum  block_config=sysgen:Accum_config  block_width=566  block_height=845
  d{1..4} (4 alike) : hdlBasic/Delay  rst=off  en=off  latency=1  reg_retiming=off  XmcBlockStatus=1  maskContainerNames=group1  block_type=delay  block_config=sysgen:Delay_config
  Envelope 2 Delay : Outport
  Envelope 4 Delay : Outport  Port=2
  Original Real : Outport  Port=3
  Original Imag : Outport  Port=4
  D2 Real : Outport  Port=5
  D2 Imag : Outport  Port=6
  D4 Real : Outport  Port=7
  D4 Imag : Outport  Port=8
  wires:
  Imag/1 -> Imag_component/1, SquareReal1/2, SquareReal1/1
  SquareReal1/1 -> SumSquares/2
  TotalSum/1 -> Display/1, Convert/1
  SumSquares/1 -> Convert6/1, TotalSum/1
  SquareReal/1 -> SumSquares/1
  Real/1 -> Real_component/1, SquareReal/1, SquareReal/2
  Valid/1 -> Delay/1
  Constant4/1 -> Mean/4
  Delay/1 -> Delay1/1
  2 TAP Envelope/1 -> Envelope 2 Delay/1
  Constant1/1 -> NoiseSampleDone/2
  Mean/3 -> Threshold_delay/1
  NoiseSampleDone/1 -> Mean/3, NOT/1, Mean/1
  Convert/1 -> Mean/2
  Delay1/1 -> Delay2/1
  NOT/1 -> AND/1, TotalSum/2
  Delay2/1 -> AND/2
  Convert6/1 -> Delay3/1
  AND/1 -> Counter/1
  Delay3/1 -> Envelope Detector/1, Display2/1
  d2/1 -> d3/1, 2 TAP Envelope/1, 4 TAP Envelope/3
  Counter/1 -> NoiseSampleDone/1
  Mean/1 -> Terminator2/1
  Mean/2 -> Terminator1/1
  Mean/4 -> Convert4/1
  Convert4/1 -> CMult/1
  CMult/1 -> Display1/1, Envelope Detector/2
  Threshold_delay/1 -> Envelope Detector/3
  d4/1 -> 4 TAP Envelope/1
  Envelope Detector/1 -> 4 TAP Envelope/5, 2 TAP Envelope/3, d1/1
  d1/1 -> 2 TAP Envelope/2, d2/1, 4 TAP Envelope/4
  d3/1 -> 4 TAP Envelope/2, d4/1
  4 TAP Envelope/1 -> Envelope 4 Delay/1
  D1/1 -> D2/1
  Real_component/1 -> Original Real/1, D1/1
  Imag_component/1 -> D1_1/1, Original Imag/1
  D1_1/1 -> D2_1/1
  D2/1 -> D3/1, D2 Real/1
  D2_1/1 -> D3_1/1, D2 Imag/1
  D3/1 -> D4/1
  D3_1/1 -> D4_1/1
  D4_1/1 -> D4 Imag/1
  D4/1 -> D4 Real/1
